simulink model "Elevator_Three_floors"  (R2024b)
settings: Solver=VariableStepAuto  StartTime=0.0  StopTime=inf  RelTol=1e-3
settings Model: Creator=ksamb  LastModifiedBy=suman

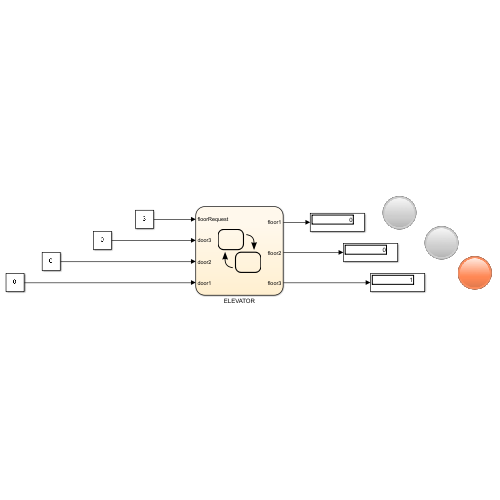
[thumbnail: Simulink's stored preview of the top-level diagram]
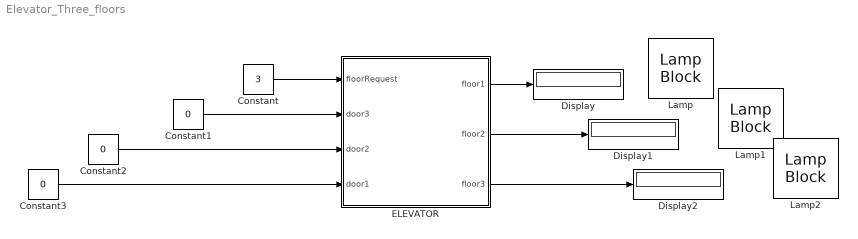
== system Elevator_Three_floors ==
  Constant : Constant  Value=3
  Constant1 : Constant  Value=0
  Constant2 : Constant  Value=0
  Constant3 : Constant  Value=0
  Display : Display
  Display1 : Display
  Display2 : Display
  ELEVATOR : Stateflow chart  TreatAsAtomicUnit=on
  Lamp : LampBlock  LabelPosition=Hide
  Lamp1 : LampBlock  LabelPosition=Hide
  Lamp2 : LampBlock  LabelPosition=Hide
  wires:
  Constant/1 -> ELEVATOR/1(floorRequest)
  Constant1/1 -> ELEVATOR/2(door3)
  Constant2/1 -> ELEVATOR/3(door2)
  Constant3/1 -> ELEVATOR/4(door1)
  ELEVATOR/1(floor1) -> Display/1
  ELEVATOR/2(floor2) -> Display1/1
  ELEVATOR/3(floor3) -> Display2/1

== stateflow chart Elevator_Three_floors/ELEVATOR ==
  state FLOOR3
    state DoorClose
      entry:
      door3==0;
      door3==1;
      floor1=0;
      floor2=0;
      floor3=1;
    (default) -> FLOOR3.DoorClose
  state FLOOR1
    state DoorClose
      entry:
      door1==0;
      door1==1;
      floor1=1;
      floor2=0;
      floor3=0;
    (default) -> FLOOR1.DoorClose
  state FLOOR2
    state DoorClose
      entry:
      door2==0;
      door2==1;
      floor1=0;
      floor2=1;
      floor3=0;
    (default) -> FLOOR2.DoorClose
  FLOOR1 -> FLOOR3 [order 2] : [floorRequest == 3 && door1==0]
  (default) -> FLOOR1
  FLOOR1 -> FLOOR2 [order 1] : [floorRequest == 2 &&...
      | door1==0]
  FLOOR3 -> FLOOR2 [order 1] : [floorRequest == 2 && door3==0]
  FLOOR2 -> FLOOR1 [order 1] : [floorRequest == 1 &&...
      |  door2==0]
  FLOOR2 -> FLOOR3 [order 2] : [floorRequest == 3 &&...
      |  door2==0]
  FLOOR3 -> FLOOR1 [order 2] : [floorRequest == 1 &&...
      |  door3==0]
  data: floorRequest input; door3 input; door2 input; door1 input; floor1 output; floor2 output; floor3 output
